simulink model "octave_bank_eq"  (R2020a)
settings: Solver=VariableStepAuto  StartTime=0.0  StopTime=100  RelTol=1e-3
libraries: audiofilters x10, simulink x10, dspsnks4 x1, dspvision x1
settings Model: Creator=samarththopaiah  LastModifiedBy=samarththopaiah

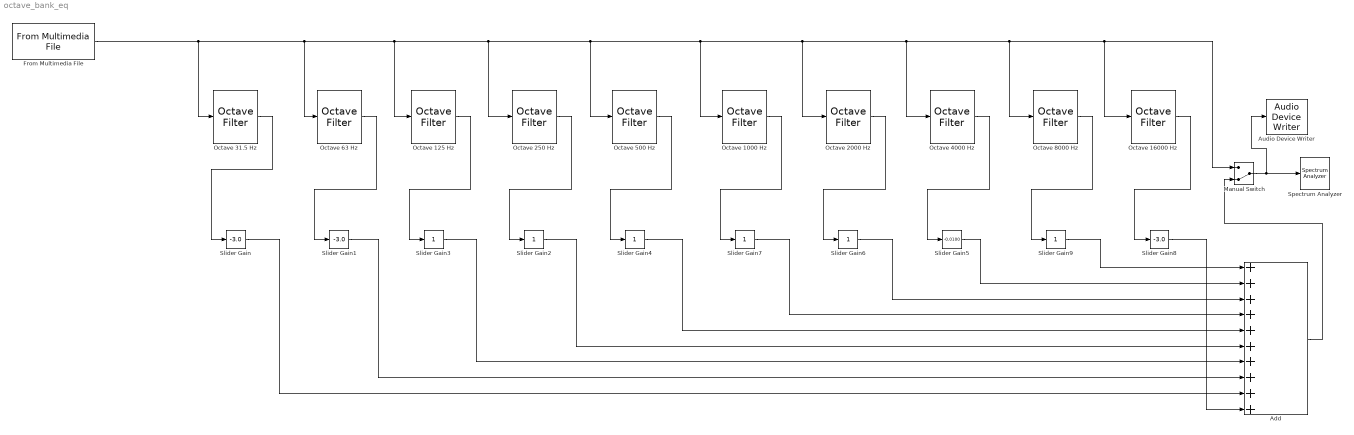
== system octave_bank_eq ==
  Add : Sum  Inputs=++++++++++
  Audio Device Writer : dspsnks4/Audio Device Writer  Driver=CoreAudio  Device=Default  InheritSampleRate=on  SampleRate=44100  BitDepth=16-bit integer  BufferSize=4096  NumBuffers=10  DefaultOutputChannelMapping=on  OutputChannelMapping=1:2  OutputNumUnderrunSamples=off  DriverIdx=5  DeviceWarnFlag=''
  From Multimedia File : dspvision/From Multimedia File  inputFilename=/Users/samarththopaiah/Desktop/Plugins/Julian-Lage-Nocturne.mp3  readRange=[1 Inf]  loop=on  numPlays=inf  outputStreams=Audio only  videoDataType=single  audioDataType=double  inheritSampleTime=on  userDefinedSampleTime=1/30  noAudioOutput=off  isIntensityVideo=off  fourcc=RGB  colorVideoFormat=Separate color signals  outputEOF=off  dataOrg=Column-major  audioFrameSize=1024  computeAudioFrameSize=off  outSamplingMode=Sample based
  Manual Switch : ManualSwitch  CurrentSetting=0
  Octave 1000 Hz : audiofilters/Octave Filter  FilterOrder=2  CenterFrequencyPort=off  CenterFrequency=1000  Bandwidth=1 octave  BandsPerOctave=1  BandwidthType=1 octave  Oversample=off  InheritSampleRate=off  SampleRate=44100  SimulateUsing=Code generation  MaskClassType=No mask
      settings: SourceProductBaseCode=AU
  Octave 125 Hz : audiofilters/Octave Filter  FilterOrder=2  CenterFrequencyPort=off  CenterFrequency=125  Bandwidth=1 octave  BandsPerOctave=1  BandwidthType=1 octave  Oversample=off  InheritSampleRate=off  SampleRate=44100  SimulateUsing=Code generation  MaskClassType=No mask
      settings: SourceProductBaseCode=AU
  Octave 16000 Hz : audiofilters/Octave Filter  FilterOrder=2  CenterFrequencyPort=off  CenterFrequency=16000  Bandwidth=1 octave  BandsPerOctave=1  BandwidthType=1 octave  Oversample=off  InheritSampleRate=off  SampleRate=44100  SimulateUsing=Code generation  MaskClassType=No mask
      settings: SourceProductBaseCode=AU
  Octave 2000 Hz : audiofilters/Octave Filter  FilterOrder=2  CenterFrequencyPort=off  CenterFrequency=4000  Bandwidth=1 octave  BandsPerOctave=1  BandwidthType=1 octave  Oversample=off  InheritSampleRate=off  SampleRate=44100  SimulateUsing=Code generation  MaskClassType=No mask
      settings: SourceProductBaseCode=AU
  Octave 250 Hz : audiofilters/Octave Filter  FilterOrder=2  CenterFrequencyPort=off  CenterFrequency=250  Bandwidth=1 octave  BandsPerOctave=1  BandwidthType=1 octave  Oversample=off  InheritSampleRate=off  SampleRate=44100  SimulateUsing=Code generation  MaskClassType=No mask
      settings: SourceProductBaseCode=AU
  Octave 31.5 Hz : audiofilters/Octave Filter  FilterOrder=2  CenterFrequencyPort=off  CenterFrequency=31.5  Bandwidth=1 octave  BandsPerOctave=1  BandwidthType=1 octave  Oversample=off  InheritSampleRate=off  SampleRate=44100  SimulateUsing=Code generation  MaskClassType=No mask
      settings: SourceProductBaseCode=AU
  Octave 4000 Hz : audiofilters/Octave Filter  FilterOrder=2  CenterFrequencyPort=off  CenterFrequency=4000  Bandwidth=1 octave  BandsPerOctave=1  BandwidthType=1 octave  Oversample=off  InheritSampleRate=off  SampleRate=44100  SimulateUsing=Code generation  MaskClassType=No mask
      settings: SourceProductBaseCode=AU
  Octave 500 Hz : audiofilters/Octave Filter  FilterOrder=2  CenterFrequencyPort=off  CenterFrequency=500  Bandwidth=1 octave  BandsPerOctave=1  BandwidthType=1 octave  Oversample=off  InheritSampleRate=off  SampleRate=44100  SimulateUsing=Code generation  MaskClassType=No mask
      settings: SourceProductBaseCode=AU
  Octave 63 Hz : audiofilters/Octave Filter  FilterOrder=2  CenterFrequencyPort=off  CenterFrequency=63  Bandwidth=1 octave  BandsPerOctave=1  BandwidthType=1 octave  Oversample=off  InheritSampleRate=off  SampleRate=44100  SimulateUsing=Code generation  MaskClassType=No mask
      settings: SourceProductBaseCode=AU
  Octave 8000 Hz : audiofilters/Octave Filter  FilterOrder=2  CenterFrequencyPort=off  CenterFrequency=8000  Bandwidth=1 octave  BandsPerOctave=1  BandwidthType=1 octave  Oversample=off  InheritSampleRate=off  SampleRate=44100  SimulateUsing=Code generation  MaskClassType=No mask
      settings: SourceProductBaseCode=AU
  Slider Gain : simulink/Math Operations/Slider Gain  gain=-3.0  low=-3  high=10
  Slider Gain1 : simulink/Math Operations/Slider Gain  gain=-3.0  low=-3  high=10
  Slider Gain{2..4,6..7,9} (6 alike) : simulink/Math Operations/Slider Gain  gain=1  low=-3  high=10
  Slider Gain5 : simulink/Math Operations/Slider Gain  gain=-0.0100  low=-3  high=10
  Slider Gain8 : simulink/Math Operations/Slider Gain  gain=-3.0  low=-3  high=10
  Spectrum Analyzer : SpectrumAnalyzer
  wires:
  Octave 2000 Hz/1 -> Slider Gain6/1
  Octave 4000 Hz/1 -> Slider Gain5/1
  Octave 8000 Hz/1 -> Slider Gain9/1
  Octave 16000 Hz/1 -> Slider Gain8/1
  Octave 1000 Hz/1 -> Slider Gain7/1
  Octave 500 Hz/1 -> Slider Gain4/1
  Octave 250 Hz/1 -> Slider Gain2/1
  Octave 125 Hz/1 -> Slider Gain3/1
  Octave 63 Hz/1 -> Slider Gain1/1
  Octave 31.5 Hz/1 -> Slider Gain/1
  From Multimedia File/1 -> Octave 63 Hz/1, Octave 125 Hz/1, Octave 250 Hz/1, Octave 500 Hz/1, Octave 1000 Hz/1, Octave 2000 Hz/1, Octave 4000 Hz/1, Octave 8000 Hz/1, Octave 16000 Hz/1, Manual Switch/1, Octave 31.5 Hz/1
  Add/1 -> Manual Switch/2
  Slider Gain/1 -> Add/9
  Slider Gain1/1 -> Add/8
  Slider Gain3/1 -> Add/7
  Slider Gain2/1 -> Add/6
  Slider Gain4/1 -> Add/5
  Slider Gain7/1 -> Add/4
  Slider Gain6/1 -> Add/3
  Slider Gain5/1 -> Add/2
  Slider Gain9/1 -> Add/1
  Slider Gain8/1 -> Add/10
  Manual Switch/1 -> Audio Device Writer/1, Spectrum Analyzer/1
